simulink model "inClassHeatedResistor"  (R2015a)
settings: Solver=ode45  StartTime=0.0  StopTime=10.0  MaxStep=.05  RelTol=1e-3
undefined symbols (not defined in the file): A, Cp, h, m
settings Model: Creator=nathan  LastModifiedBy=nathan

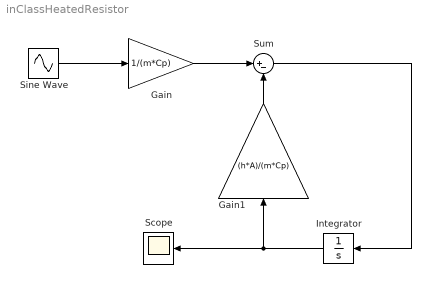
== system inClassHeatedResistor ==
  Gain : Gain  Gain=1/(m*Cp)
  Gain1 : Gain  Gain=(h*A)/(m*Cp)
  Integrator : Integrator  InitialCondition=-10
  Scope : Scope
  Sine Wave : Sin  SampleTime=0
  Sum : Sum  Inputs=|+-
  wires:
  Integrator/1 -> Scope/1, Gain1/1
  Gain1/1 -> Sum/2
  Gain/1 -> Sum/1
  Sum/1 -> Integrator/1
  Sine Wave/1 -> Gain/1
